simulink model "Ex_1_Hall_Effect_Encoder"  (R2020a)
settings: Solver=FixedStepAuto  StartTime=0.0  StopTime=5  FixedStep=0.0001  RelTol=1e-3
values from neighbouring files (symbols this model uses):
  J = 0.005    [motor_parameters.mat]
  Ke = 2.3    [motor_parameters.mat]
  Kf = 0.3    [motor_parameters.mat]
  Kt = 2.19    [motor_parameters.mat]
  L = 1    [motor_parameters.mat]
  R = 1.1    [motor_parameters.mat]
libraries: fl_lib x9, ee_lib x6, nesl_utility x6
settings Model: Creator=alexr  LastModifiedBy=alexr

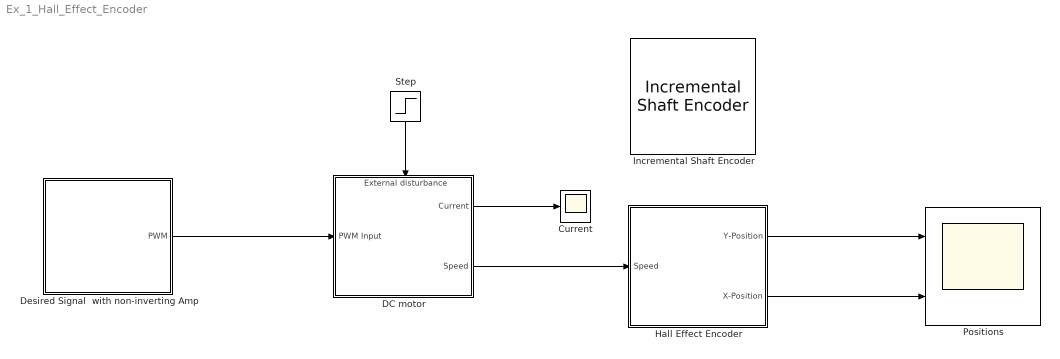
== system Ex_1_Hall_Effect_Encoder ==
  Current : Scope
  DC motor : Subsystem
      settings: PortSchema="{\"entries\":[{\"content\":{\"sides\":[{\"content\":{\"connectorIds\":[\"In1\"]},\"type\":\"ConnectorPlacement.EquallySpacedRectSide\",\"uuid\":\"b8964f03-f732-4eca-8bb3-271c6a142913\"},{\"content\":{\"connectorIds\":[\"Out1\",\"Out2\"],\"side\":\"RIGHT\"},\"type\":\"ConnectorPlacement.EquallySpacedRectSide\",\"uuid\":\"d9454742-672e-4fe5-95f0-bbd13d54c419\"},{\"content\":{\"connectorIds\":[\"In2\"],\"side\":\"TOP\"},\"type\":\"ConnectorPlacement.EquallySpacedRectSide\",\"uuid\":\"e6caae02-41c3-4a6e-bc88-5a1dbae17927\"}]},\"type\":\"ConnectorPlacement.EquallySpacedConnector\",\"uuid\":\"63b5fd96-b4f9-40de-b12b-448e4637e2c5\"}],\"packageUris\":[\"http://schema.mathworks.com/mf0/Connector/19700101\"],\"version\":\"1.0\"}"
  Desired Signal  with non-inverting Amp : Subsystem
  Hall Effect Encoder : Subsystem
  Incremental Shaft Encoder : ee_lib/Sensors & Transducers/Incremental Shaft Encoder  NPulse=2  Vm=5 V  angle0=0 deg
      settings: SourceProductBaseCode=PS  InternalSimscapePortConfiguration="{\"Bottom\":[],\"Left\":[{\"id\":\"R\",\"label\":\"R\",\"type\":\"foundation.mechanical.rotational.rotational\"},{\"id\":\"C\",\"label\":\"C\",\"type\":\"foundation.mechanical.rotational.rotational\"}],\"Right\":[{\"id\":\"A\",\"label\":\"A\",\"type\":\"foundation.electrical.electrical\"},{\"id\":\"B\",\"label\":\"B\",\"type\":\"foundation.electrical.electrical\"},{\"id\":\"Z\",\"label\":\"Z\",\"type\":\"foundation.electrical.electrical\"},{\"id\":\"GND\",\"label\":\"REF\",\"type\":\"foundation.electrical.electrical\"}],\"Top\":[]}"
  Positions : Scope  NumInputPorts=2
  "Step " : Step  Time=5  After=0  SampleTime=0
  wires:
  "Step "/1 -> DC motor/2(External disturbance)
  DC motor/1(Current) -> Current/1
  Desired Signal  with non-inverting Amp/1(PWM) -> DC motor/1(PWM Input)
  DC motor/2(Speed) -> Hall Effect Encoder/1(Speed)
  Hall Effect Encoder/1(Y-Position) -> Positions/1
  Hall Effect Encoder/2(X-Position) -> Positions/2

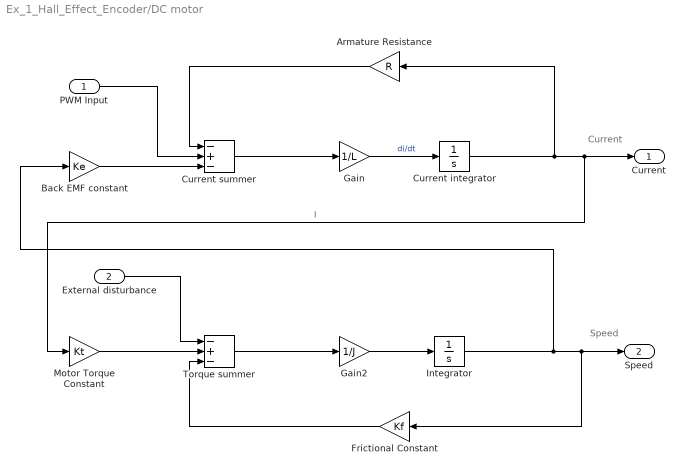
== system Ex_1_Hall_Effect_Encoder/DC motor ==
  note: Speed
  note: Current
  PWM Input : Inport
  External disturbance : Inport  Port=2
  Armature Resistance : Gain  Gain=R
  Back EMF constant : Gain  Gain=Ke
  Current integrator : Integrator
  Current summer : Sum  Inputs=-+-
  Frictional Constant : Gain  Gain=Kf
  Gain : Gain  Gain=1/L
  Gain2 : Gain  Gain=1/J
  Integrator : Integrator
  Motor Torque Constant : Gain  Gain=Kt
  Torque summer : Sum  Inputs=-+-
  Current : Outport
  Speed : Outport  Port=2
  wires:
  Current summer/1 -> Gain/1
  Gain2/1 -> Integrator/1
  Integrator/1 -> Back EMF constant/1, Speed/1, Frictional Constant/1
  Torque summer/1 -> Gain2/1
  Armature Resistance/1 -> Current summer/1
  PWM Input/1 -> Current summer/2
  Gain/1 -> Current integrator/1  "di/dt"
  Motor Torque Constant/1 -> Torque summer/2
  External disturbance/1 -> Torque summer/1
  Frictional Constant/1 -> Torque summer/3
  Current integrator/1 -> Armature Resistance/1, Current/1, Motor Torque Constant/1  "I"
  Back EMF constant/1 -> Current summer/3

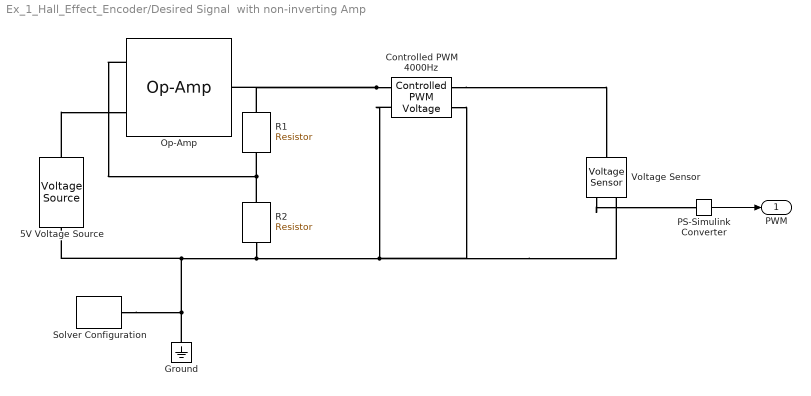
== system Ex_1_Hall_Effect_Encoder/Desired Signal  with non-inverting Amp ==
  "5V Voltage Source " : ee_lib/Sources/Voltage Source  dc_voltage=5 V  ac_voltage=0 V  ac_shift=0 rad  ac_frequency=60 Hz  noise_mode=0  PSD=0 V^2/Hz  repeatability=1  auto_seed=2868319722  user_seed=0  sample_time=1e-3 s  i_specify=off  i_priority=None  i=0 A  i_nominal_specify=off  i_nominal_unit=A  i_nominal_value=1  v_specify=off  v_priority=None  v=0 V  v_nominal_specify=off  v_nominal_unit=V  v_nominal_value=1
  "Controlled PWM 4000Hz " : ee_lib/Integrated Circuits/Controlled PWM Voltage  F=4000 Hz  TD=0 s  pulse_width_offset=0 s  pulse_min=0 s  Vmin=0 V  Vmax=10 V  Vm=10 V  pwm_or_av=2  event_type=1  sample_time=1e-6 s  u_min=0  u_max=5
  "Ground " : fl_lib/Electrical/Electrical Elements/Electrical Reference
      settings: SourceProductBaseCode=MT,SS
  "Op-Amp " : fl_lib/Electrical/Electrical Elements/Op-Amp  outI_specify=off  outI_priority=None  outI=0 A  outI_nominal_specify=off  outI_nominal_unit=A  outI_nominal_value=1
  PS-Simulink Converter : nesl_utility/PS-Simulink Converter  PhysicalDomain=network_engine_domain  SubClassName=ps_output  LeftPortType=input  RightPortType=output  PseudoPeriodic=off  Frequencies=[]  Unit=inherit  AffineConversion=off
  R1 : ee_lib/Passive/Resistor  R=1000 Ohm  R_tol=5  enable_R_tol=0  tol_distribution=1  nSigma=4  enable_operating_limits=0  operating_limit_action=2  max_working_voltage=100 V  power_rating=1 W  enable_faults=0  fault_action=1  R_faulted=inf Ohm  enable_temporal_fault=0  t_fault=1 s  enable_behavioral_fault=0  max_permissible_current=1 A  t_fail_on_current=1 s  noise_mode=0  sample_time=1e-3 s  repeatability=1  auto_seed=3626636697  user_seed=0  Tdevice=25 degC  alpha=3.93e-3 1/K  Tmeas=25 degC  thermal_mass=100 J/K  power_derating_T1=70 degC  power_derating_T2=155 degC  operating_temperature_range_vec=[-50, 150] degC  temperature_specify=off  temperature_priority=High  temperature=298.15 K  temperature_nominal_specify=off  temperature_nominal_unit=K  temperature_nominal_value=1
  R2 : ee_lib/Passive/Resistor  R=1000 Ohm  R_tol=5  enable_R_tol=0  tol_distribution=1  nSigma=4  enable_operating_limits=0  operating_limit_action=2  max_working_voltage=100 V  power_rating=1 W  enable_faults=0  fault_action=1  R_faulted=inf Ohm  enable_temporal_fault=0  t_fault=1 s  enable_behavioral_fault=0  max_permissible_current=1 A  t_fail_on_current=1 s  noise_mode=0  sample_time=1e-3 s  repeatability=1  auto_seed=1479454791  user_seed=0  Tdevice=25 degC  alpha=3.93e-3 1/K  Tmeas=25 degC  thermal_mass=100 J/K  power_derating_T1=70 degC  power_derating_T2=155 degC  operating_temperature_range_vec=[-50, 150] degC  temperature_specify=off  temperature_priority=High  temperature=298.15 K  temperature_nominal_specify=off  temperature_nominal_unit=K  temperature_nominal_value=1
  "Solver Configuration " : nesl_utility/Solver Configuration  PhysicalDomain=network_engine_domain  SubClassName=solver  LeftPortType=input  RightPortType=generic  Tones=[]  Harmonics=[]  SimulateNoise=off  Profile=off  UseLocalSampling=off  EnableSwitchedLinearOptims=on  FrequencyDomain=off  UseCCode=off  RelTol=0.001  AbsTol=1e-06  MinStep=1e-09  ToWorkspace=off  RevertToSquareIcSolve=off  NumHomotopyIterations=100  PhasorMode=off  PhasorModeNumHarmonics=1  DoDC=off  ResidualTolerance=1e-09  UseLocalSolver=off  LocalSolverChoice=NE_BACKWARD_EULER_ADVANCER  LocalSolverSampleTime=0.001  DoFixedCost=off  MaxNonlinIter=3  MaxModeIter=2  LinearAlgebra=auto  EquationFormulation=NE_TIME_EF  DelaysMemoryBudget=1024  AutomaticFiltering=on  FilteringTimeConstant=0.001  PartitionStorageMethod=AS_NEEDED  PartitionMemoryBudget=1024  PartitionMethod=ROBUST
  Voltage Sensor : fl_lib/Electrical/Electrical Sensors/Voltage Sensor
  PWM : Outport
  wires:
  PS-Simulink Converter/1 -> PWM/1
  connections:
  R2/LConn1 -- "Op-Amp "/LConn2 -- R1/RConn1
  "Controlled PWM 4000Hz "/LConn1 -- "Op-Amp "/RConn1 -- R1/LConn1
  "Solver Configuration "/RConn1 -- "Ground "/LConn1 -- R2/RConn1 -- Voltage Sensor/RConn2 -- "Controlled PWM 4000Hz "/RConn2 -- "Controlled PWM 4000Hz "/LConn2 -- "5V Voltage Source "/RConn1
  "5V Voltage Source "/LConn1 -- "Op-Amp "/LConn1
  "Controlled PWM 4000Hz "/RConn1 -- Voltage Sensor/LConn1
  Voltage Sensor/RConn1 -- PS-Simulink Converter/LConn1

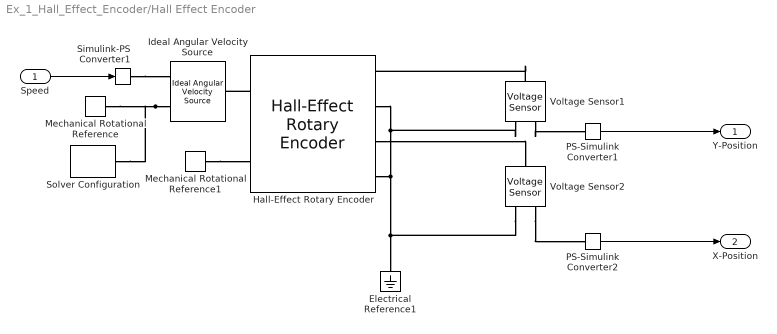
== system Ex_1_Hall_Effect_Encoder/Hall Effect Encoder ==
  Speed : Inport
  Electrical Reference1 : fl_lib/Electrical/Electrical Elements/Electrical Reference
      settings: SourceProductBaseCode=MT,SS
  "Hall-Effect Rotary Encoder " : ee_lib/Sensors & Transducers/Hall-Effect Rotary Encoder  Ax=10 V  Ay=10 V  Vx0=0 V  Vy0=0 V  beta=0 deg  sensor_output=ee.enum.rotarysensors.output.elec  theta_specify=off  theta_priority=High  theta=0 deg  theta_nominal_specify=off  theta_nominal_unit=deg  theta_nominal_value=1
      settings: SourceProductBaseCode=PS  InternalSimscapePortConfiguration="{\"Bottom\":[],\"Left\":[{\"id\":\"R\",\"label\":\"R\",\"type\":\"foundation.mechanical.rotational.rotational\"},{\"id\":\"C\",\"label\":\"C\",\"type\":\"foundation.mechanical.rotational.rotational\"}],\"Right\":[{\"id\":\"yp\",\"label\":\"yp\",\"type\":\"foundation.electrical.electrical\"},{\"id\":\"yn\",\"label\":\"yn\",\"type\":\"foundation.electrical.electrical\"},{\"id\":\"xp\",\"label\":\"xp\",\"type\":\"foundation.electrical.electrical\"},{\"id\":\"xn\",\"label\":\"xn\",\"type\":\"foundation.electrical.electrical\"}],\"Top\":[]}"
  "Ideal Angular Velocity Source " : fl_lib/Mechanical/Mechanical Sources/Ideal Angular Velocity Source
  Mechanical Rotational Reference : fl_lib/Mechanical/Rotational Elements/Mechanical Rotational Reference
  Mechanical Rotational Reference1 : fl_lib/Mechanical/Rotational Elements/Mechanical Rotational Reference
  PS-Simulink Converter1 : nesl_utility/PS-Simulink Converter  PhysicalDomain=network_engine_domain  SubClassName=ps_output  LeftPortType=input  RightPortType=output  PseudoPeriodic=off  Frequencies=[]  Unit=inherit  AffineConversion=off
  PS-Simulink Converter2 : nesl_utility/PS-Simulink Converter  PhysicalDomain=network_engine_domain  SubClassName=ps_output  LeftPortType=input  RightPortType=output  PseudoPeriodic=off  Frequencies=[]  Unit=inherit  AffineConversion=off
  Simulink-PS Converter1 : nesl_utility/Simulink-PS Converter  PhysicalDomain=network_engine_domain  SubClassName=ps_input  LeftPortType=input  RightPortType=output  PseudoPeriodic=off  Frequencies=[]  NoiseDistribution=none  NoiseParameters=[]  Unit=1  AffineConversion=off  FilteringAndDerivatives=provide  SimscapeFilterOrder=1  InputFilterTimeConstant=0.001  UdotUserProvided=0
  "Solver Configuration " : nesl_utility/Solver Configuration  PhysicalDomain=network_engine_domain  SubClassName=solver  LeftPortType=input  RightPortType=generic  Tones=[]  Harmonics=[]  SimulateNoise=off  Profile=off  UseLocalSampling=off  EnableSwitchedLinearOptims=on  FrequencyDomain=off  UseCCode=off  RelTol=0.001  AbsTol=1e-06  MinStep=1e-09  ToWorkspace=off  RevertToSquareIcSolve=off  NumHomotopyIterations=100  PhasorMode=off  PhasorModeNumHarmonics=1  DoDC=off  ResidualTolerance=1e-09  UseLocalSolver=off  LocalSolverChoice=NE_BACKWARD_EULER_ADVANCER  LocalSolverSampleTime=0.001  DoFixedCost=off  MaxNonlinIter=3  MaxModeIter=2  LinearAlgebra=auto  EquationFormulation=NE_TIME_EF  DelaysMemoryBudget=1024  AutomaticFiltering=on  FilteringTimeConstant=0.001  PartitionStorageMethod=AS_NEEDED  PartitionMemoryBudget=1024  PartitionMethod=ROBUST
  Voltage Sensor1 : fl_lib/Electrical/Electrical Sensors/Voltage Sensor
  Voltage Sensor2 : fl_lib/Electrical/Electrical Sensors/Voltage Sensor
  Y-Position : Outport
  X-Position : Outport  Port=2
  wires:
  Speed/1 -> Simulink-PS Converter1/1
  PS-Simulink Converter2/1 -> X-Position/1
  PS-Simulink Converter1/1 -> Y-Position/1
  connections:
  Voltage Sensor1/RConn2 -- "Hall-Effect Rotary Encoder "/RConn2 -- "Hall-Effect Rotary Encoder "/RConn4 -- Voltage Sensor2/RConn2 -- Electrical Reference1/LConn1
  "Ideal Angular Velocity Source "/RConn2 -- Mechanical Rotational Reference/LConn1 -- "Solver Configuration "/RConn1
  Voltage Sensor1/LConn1 -- "Hall-Effect Rotary Encoder "/RConn1
  "Hall-Effect Rotary Encoder "/RConn3 -- Voltage Sensor2/LConn1
  Voltage Sensor2/RConn1 -- PS-Simulink Converter2/LConn1
  Mechanical Rotational Reference1/LConn1 -- "Hall-Effect Rotary Encoder "/LConn2
  Simulink-PS Converter1/RConn1 -- "Ideal Angular Velocity Source "/RConn1
  "Hall-Effect Rotary Encoder "/LConn1 -- "Ideal Angular Velocity Source "/LConn1
  Voltage Sensor1/RConn1 -- PS-Simulink Converter1/LConn1
